simulink subsystem "Battery"  (R2022a)
settings: Solver=VariableStepAuto  StartTime=0.0  StopTime=10.0  RelTol=1e-3
undefined symbols (not defined in the file or in its folder): Neg, Pos
settings Model: Creator=mmarq  LastModifiedBy=mmarq

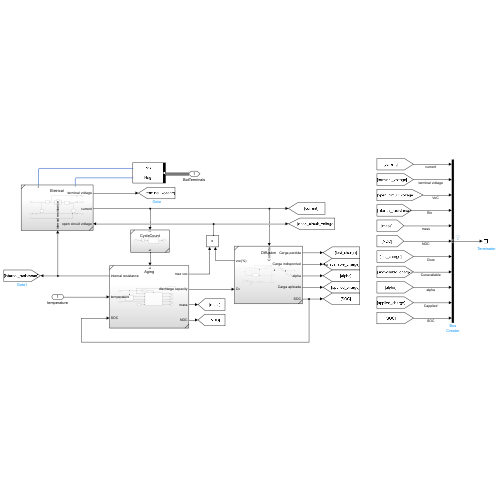
[thumbnail: Simulink's stored preview of the top-level diagram]
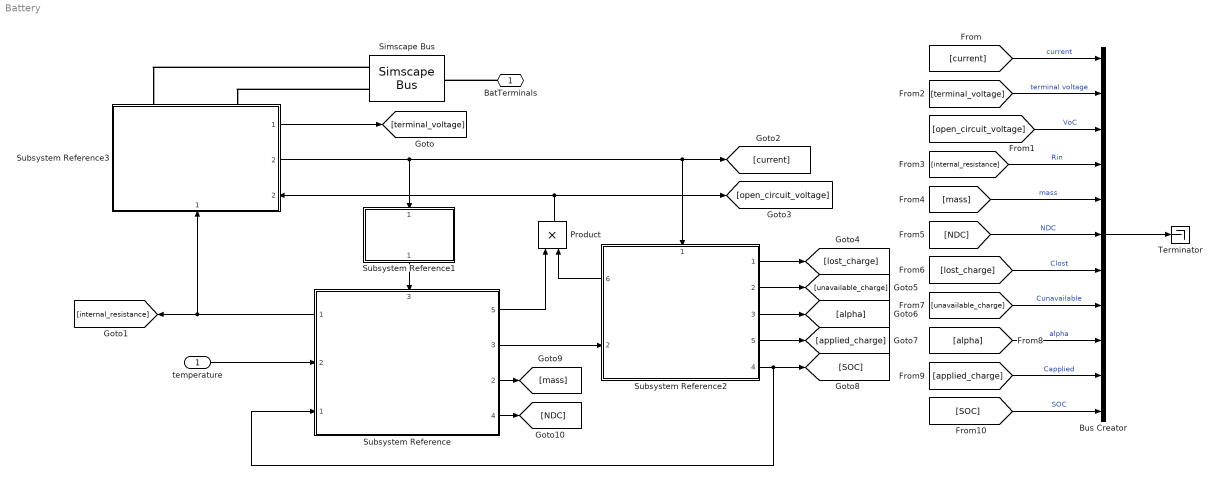
== system Battery ==
  temperature : Inport
  Bus Creator : BusCreator  Inputs=11
  Product : Product
  Simscape Bus : SimscapeBus  HierarchyStrings=Pos;Neg
  Subsystem Reference : Subsystem  ReferencedSubsystem=Aging
      settings: PortSchema="{\"entries\":[{\"content\":{\"sides\":[{\"content\":{\"connectorIds\":[\"Out1\",\"In2\",\"In1\"]},\"type\":\"ConnectorPlacement.EquallySpacedRectSide\",\"uuid\":\"b83966b6-0d43-4123-bff6-7e6404950e83\"},{\"content\":{\"connectorIds\":[\"Out5\",\"Out3\",\"Out2\",\"Out4\"],\"side\":\"RIGHT\"},\"type\":\"ConnectorPlacement.EquallySpacedRectSide\",\"uuid\":\"3a818dd6-c1ca-422f-870c-95b34f7153d0\"},{\"content\":{\"connectorIds\":[\"In3\"],\"side\":\"TOP\"},\"type\":\"ConnectorPlacement.EquallySpacedRectSide\",\"uuid\":\"adecc11b-bd29-4b12-a0af-ab84e0c8bcdf\"}]},\"type\":\"ConnectorPlacement.EquallySpacedConnector\",\"uuid\":\"a9e16b39-9e5b-4fac-a3aa-35472259cec1\"}],\"packageUris\":[\"http://schema.mathworks.com/mf0/Connector/R2020b\"],\"version\":\"1.0\"}"
  Subsystem Reference1 : Subsystem  ReferencedSubsystem=CycleCount
      settings: PortSchema="{\"entries\":[{\"content\":{\"sides\":[{\"content\":{\"connectorIds\":[]},\"type\":\"ConnectorPlacement.EquallySpacedRectSide\",\"uuid\":\"0f8506b1-c558-4b53-9b84-b54b4f133099\"},{\"content\":{\"connectorIds\":[],\"side\":\"RIGHT\"},\"type\":\"ConnectorPlacement.EquallySpacedRectSide\",\"uuid\":\"0c238bed-9bcf-499f-b949-06a843e9a6cc\"},{\"content\":{\"connectorIds\":[\"In1\"],\"side\":\"TOP\"},\"type\":\"ConnectorPlacement.EquallySpacedRectSide\",\"uuid\":\"4925469a-a1de-48f5-a3ee-e0cd87b78795\"},{\"content\":{\"connectorIds\":[\"Out1\"],\"side\":\"BOTTOM\"},\"type\":\"ConnectorPlacement.EquallySpacedRectSide\",\"uuid\":\"e0aa39f3-eec7-4123-a08f-cdf30320134c\"}]},\"type\":\"ConnectorPlacement.EquallySpacedConnector\",\"uuid\":\"95810199-f4ed-42f7-878e-11f3bff63c1f\"}],\"packageUris\":[\"http://schema.mathworks.com/mf0/Connector/R2020b\"],\"version\":\"1.0\"}"
  Subsystem Reference2 : Subsystem  ReferencedSubsystem=Diffusion
      settings: PortSchema="{\"entries\":[{\"content\":{\"sides\":[{\"content\":{\"connectorIds\":[\"Out6\",\"In2\"]},\"type\":\"ConnectorPlacement.EquallySpacedRectSide\",\"uuid\":\"2175449e-25ad-4a14-852b-b8fec13c56eb\"},{\"content\":{\"connectorIds\":[\"Out1\",\"Out2\",\"Out3\",\"Out5\",\"Out4\"],\"side\":\"RIGHT\"},\"type\":\"ConnectorPlacement.EquallySpacedRectSide\",\"uuid\":\"9ef1a6f0-1215-4e70-af05-ca65aa15645f\"},{\"content\":{\"connectorIds\":[\"In1\"],\"side\":\"TOP\"},\"type\":\"ConnectorPlacement.EquallySpacedRectSide\",\"uuid\":\"6814a118-23d0-412a-90d1-e060a452933a\"}]},\"type\":\"ConnectorPlacement.EquallySpacedConnector\",\"uuid\":\"027f8b58-52de-40a3-bf42-f9de2122c061\"}],\"packageUris\":[\"http://schema.mathworks.com/mf0/Connector/R2020b\"],\"version\":\"1.0\"}"
  Subsystem Reference3 : Subsystem  ReferencedSubsystem=Eletrical
      settings: PortSchema="{\"entries\":[{\"content\":{\"sides\":[{\"content\":{\"connectorIds\":[]},\"type\":\"ConnectorPlacement.EquallySpacedRectSide\",\"uuid\":\"cf1e1e4e-7143-45ab-a874-4d9cc96d9a12\"},{\"content\":{\"connectorIds\":[\"Out1\",\"Out2\",\"In2\"],\"side\":\"RIGHT\"},\"type\":\"ConnectorPlacement.EquallySpacedRectSide\",\"uuid\":\"18451c83-2cc0-42a3-bbbc-0880116e95f6\"},{\"content\":{\"connectorIds\":[\"LConn1\",\"LConn2\"],\"side\":\"TOP\"},\"type\":\"ConnectorPlacement.EquallySpacedRectSide\",\"uuid\":\"197d5e67-08be-498c-949c-2c9446ef6afd\"},{\"content\":{\"connectorIds\":[\"In1\"],\"side\":\"BOTTOM\"},\"type\":\"ConnectorPlacement.EquallySpacedRectSide\",\"uuid\":\"66f29f25-6101-41f6-ba60-3f471a3d501a\"}]},\"type\":\"ConnectorPlacement.EquallySpacedConnector\",\"uuid\":\"a14eea88-3bea-42bf-9c6e-73fab754c8a8\"}],\"packageUris\":[\"http://schema.mathworks.com/mf0/Connector/R2020b\"],\"version\":\"1.0\"}"
  Terminator : Terminator
  BatTerminals : PMIOPort  Side=Left
  wires:
  Subsystem Reference1/1 -> Subsystem Reference/3
  Subsystem Reference/5 -> Product/1
  Subsystem Reference2/6 -> Product/2
  Product/1 -> [open_circuit_voltage], Subsystem Reference3/2
  Subsystem Reference/3 -> Subsystem Reference2/2
  Subsystem Reference/1 -> [internal_resistance], Subsystem Reference3/1
  Subsystem Reference2/4 -> [SOC], Subsystem Reference/1
  Subsystem Reference3/2 -> Subsystem Reference1/1, [current], Subsystem Reference2/1
  temperature/1 -> Subsystem Reference/2
  Subsystem Reference3/1 -> [terminal_voltage]
  Subsystem Reference2/1 -> [lost_charge]
  Subsystem Reference2/2 -> [unavailable_charge]
  Subsystem Reference2/3 -> [alpha]
  Subsystem Reference2/5 -> [applied_charge]
  Subsystem Reference/2 -> [mass]
  Subsystem Reference/4 -> [NDC]
  [current] -> Bus Creator/1  "current"
  [terminal_voltage] -> Bus Creator/2  "terminal voltage"
  [open_circuit_voltage] -> Bus Creator/3  "VoC"
  [internal_resistance] -> Bus Creator/4  "Rin"
  [mass] -> Bus Creator/5  "mass"
  [NDC] -> Bus Creator/6  "NDC"
  [lost_charge] -> Bus Creator/7  "Clost"
  [unavailable_charge] -> Bus Creator/8  "Cunavailable"
  [alpha] -> Bus Creator/9  "alpha"
  [applied_charge] -> Bus Creator/10  "Capplied"
  [SOC] -> Bus Creator/11  "SOC"
  Bus Creator/1 -> Terminator/1
  connections:
  Simscape Bus/LConn1 -- Subsystem Reference3/LConn1
  Simscape Bus/LConn2 -- Subsystem Reference3/LConn2
  BatTerminals/RConn1 -- Simscape Bus/RConn1
